simulink model "audio_model"  (R2019a)
settings: Solver=VariableStepAuto  StartTime=0.0  StopTime=inf  RelTol=1e-3
InitFcn:
  | load nummat;
values from neighbouring files (symbols this model uses):
  nummat = [0.000231964447521 0.00104709389408 0.000124293590629 -0.00152411529578 0.00149987312751 -0.00100771934553 0.000227854693556 0.000793885157085 0.000295001022433 -7.66359312897e-05 0.00152762640585 -0.00116029130411 ... (512 elements, 8x64)]    [nummat.mat]
libraries: dspsnks4 x1, dspvision x1, simulink x1, dspindex x1
settings Model: Creator=Marat  LastModifiedBy=Marat

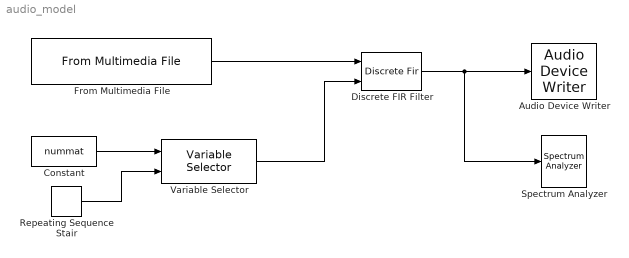
== system audio_model ==
  Audio Device Writer : dspsnks4/Audio Device Writer  Driver=DirectSound  Device=Default  InheritSampleRate=on  SampleRate=44100  BitDepth=16-bit integer  BufferSize=4096  NumBuffers=10  DefaultOutputChannelMapping=on  OutputChannelMapping=1:2  OutputNumUnderrunSamples=off  DriverIdx=1  DeviceWarnFlag=''
  Constant : Constant  Value=nummat
  Discrete FIR Filter : DiscreteFir  CoefSource=Input port  InputProcessing=Columns as channels (frame based)
      settings: InputPortMap=u0,u1
  From Multimedia File : dspvision/From Multimedia File  inputFilename=D:\Work\MainDemos\DSP\examples\DSP_YoutubePlaylist\deploy\dance.mp3  readRange=[1 Inf]  loop=on  numPlays=inf  outputStreams=Audio only  videoDataType=single  audioDataType=double  inheritSampleTime=on  userDefinedSampleTime=1/30  noAudioOutput=off  isIntensityVideo=off  fourcc=RGB  colorVideoFormat=Separate color signals  outputEOF=off  dataOrg=Column-major  audioFrameSize=4410  computeAudioFrameSize=off  outSamplingMode=Sample based
      settings: SourceProductName=DSP System Toolbox  SourceProductBaseCode=DS
  Repeating Sequence Stair : simulink/Sources/Repeating Sequence Stair  OutValues=[1 2 3 4 5 6 7 8 7 6 5 4 3 2]  tsamp=0.1  OutMin=[]  OutMax=[]  OutDataTypeStr=double  OutputDataTypeScalingMode=double  OutDataType=fixdt(0,8)  ConRadixGroup=Best Precision: Vector-wise  OutScaling=2^-12
  Spectrum Analyzer : SpectrumAnalyzer
  Variable Selector : dspindex/Variable Selector  NumInputs=1  rowsOrCols=Rows  IdxMode=Variable  Elements=[1 3]  ZerOneIdxMode=One-based  errmode=Clip Index  FillMode=on  FillValues=0
  wires:
  From Multimedia File/1 -> Discrete FIR Filter/1
  Discrete FIR Filter/1 -> Spectrum Analyzer/1, Audio Device Writer/1
  Constant/1 -> Variable Selector/1
  Variable Selector/1 -> Discrete FIR Filter/2
  Repeating Sequence Stair/1 -> Variable Selector/2
